simulink model "sampleModel1914"  (R2023a)
settings: Solver=VariableStepAuto  StartTime=0.0  StopTime=10.0  RelTol=1e-3
libraries: hdlsllib x3, simulink x2
settings Model: Creator=user1  LastModifiedBy=user1

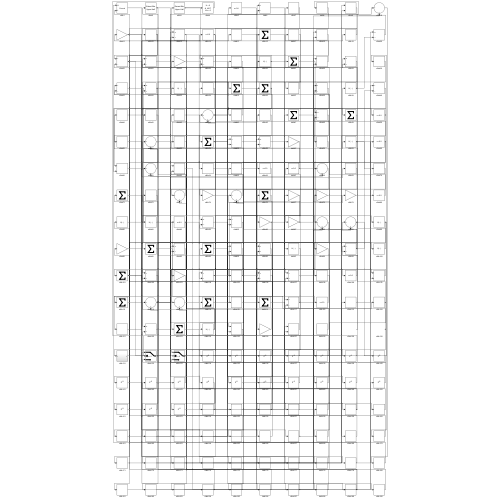
[thumbnail: Simulink's stored preview of the top-level diagram]
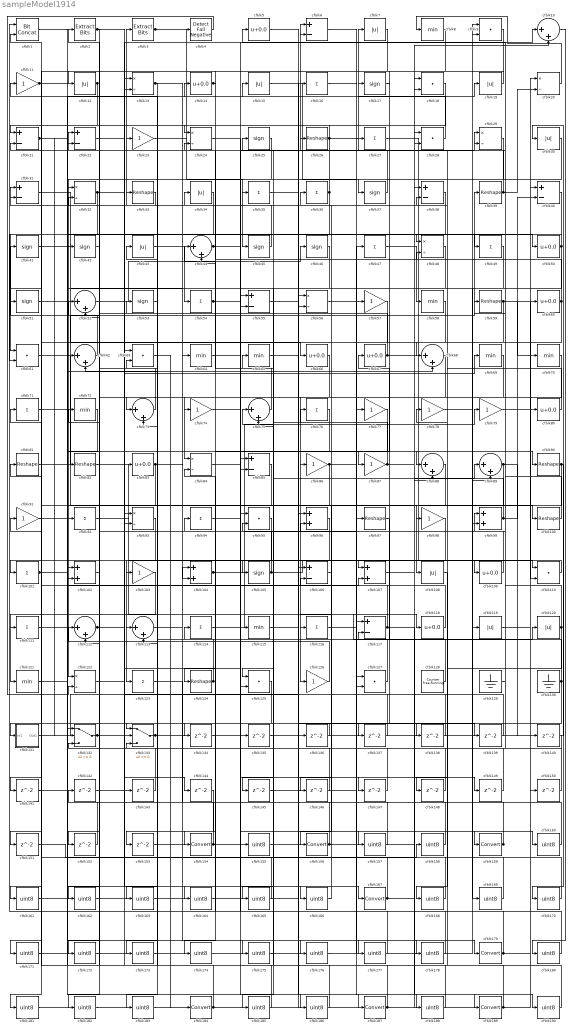
== system sampleModel1914 ==
  cfblk1 : hdlsllib/Logic and Bit Operations/Bit Concat  numInputs=2
  cfblk{10,44,52,62,68,73,75,88..89,112..113} (11 alike) : Sum  Inputs=|++
  cfblk{26,33,39,59,81..82,90,97,100,124} (10 alike) : Reshape
  cfblk{16,27,35..36,47,49,54,71,76,92,94,101,111,114,116,123} (16 alike) : Sum  Inputs=+
  cfblk{96,99,102,104,107} (5 alike) : Sum
  cfblk{11,23,57,74,77..79,86..87,91,98,103,126} (13 alike) : Gain
  cfblk{17,25,37,41..42,45..46,51,53,105} (10 alike) : Signum
  cfblk{6,21..22,31,38,40,55,85,106,117} (10 alike) : Sum  Inputs=+-
  cfblk{7,12,15,19,30,34,43,108,119..120} (10 alike) : Abs  SaturateOnIntegerOverflow=off
  cfblk{5,14,50,60,66..67,80,83,109,118} (10 alike) : Bias  Bias=0.0  SaturateOnIntegerOverflow=off
  cfblk{9,18,28,61,63,95,110,125,127} (9 alike) : DotProduct  OutDataTypeStr=Inherit: Inherit via internal rule
  cfblk{8,58,64..65,69..70,72,115,121} (9 alike) : MinMax
  cfblk{13,20,24,29,32,48,56,84,93,122} (10 alike) : Product  Inputs=*/  RndMeth=Zero  SaturateOnIntegerOverflow=on
  cfblk128 : hdlsllib/Sources/Counter Free-Running  NumBits=16  tsamp=-1
  cfblk129 : Ground
  cfblk130 : Ground
  cfblk131 : Subsystem
      settings: LibrarySourceBlock=|
      | hdlsllib/Ports &
      | Subsystems/Subsystem
  cfblk132 : Switch  SaturateOnIntegerOverflow=off  InputSameDT=off
  cfblk133 : Switch  SaturateOnIntegerOverflow=off  InputSameDT=off
  cfblk{134..153} (20 alike) : Delay  SampleTime=1
  cfblk{154,156,159,167,179,184,187,189} (8 alike) : DataTypeConversion  SaturateOnIntegerOverflow=off  RndMeth=Floor
  cfblk{155,157..158,160..166,168..178,180..183,185..186,188,190} (29 alike) : DataTypeConversion  OutDataTypeStr=uint8  SaturateOnIntegerOverflow=off  RndMeth=Floor
  cfblk2 : simulink/Logic and Bit Operations/Extract Bits  bitsToExtract=Upper half  numBits=8  bitIdxRange=[0 7]  outScalingMode=Preserve fixed-point scaling
      settings: LibrarySourceBlock=|
      | hdlsllib/Logic and Bit
      | Operations/Extract Bits
  cfblk3 : simulink/Logic and Bit Operations/Extract Bits  bitsToExtract=Upper half  numBits=8  bitIdxRange=[0 7]  outScalingMode=Preserve fixed-point scaling
      settings: LibrarySourceBlock=|
      | hdlsllib/Logic and Bit
      | Operations/Extract Bits
  cfblk4 : hdlsllib/Logic and Bit Operations/Detect Fall Negative  vinit=0  OutDataTypeStr=boolean
  wires:
  cfblk83/1 -> cfblk105/1, cfblk182/1
  cfblk105/1 -> cfblk107/1, cfblk72/1
  cfblk86/1 -> cfblk117/1, cfblk151/1
  cfblk19/1 -> cfblk12/1
  cfblk82/1 -> cfblk120/1
  cfblk104/1 -> cfblk79/1, cfblk84/2
  cfblk106/1 -> cfblk156/1
  cfblk130/1 -> cfblk67/1, cfblk183/1
  cfblk66/1 -> cfblk126/1
  cfblk94/1 -> cfblk179/1
  cfblk45/1 -> cfblk3/1
  cfblk46/1 -> cfblk125/1
  cfblk72/1 -> cfblk122/1
  cfblk67/1 -> cfblk109/1, cfblk31/2
  cfblk30/1 -> cfblk45/1
  cfblk103/1 -> cfblk121/1
  cfblk114/1 -> cfblk47/1
  cfblk25/1 -> cfblk92/1
  cfblk37/1 -> cfblk7/1
  cfblk27/1 -> cfblk100/1
  cfblk3/1 -> cfblk35/1, cfblk4/1
  cfblk92/1 -> cfblk110/1
  cfblk99/1 -> cfblk25/1, cfblk24/2, cfblk40/2
  cfblk40/1 -> cfblk61/1
  cfblk5/1 -> cfblk96/1
  cfblk12/1 -> cfblk21/1, cfblk51/1
  cfblk61/1 -> cfblk108/1
  cfblk93/1 -> cfblk123/1
  cfblk20/1 -> cfblk8/1
  cfblk31/1 -> cfblk66/1
  cfblk6/1 -> cfblk27/1
  cfblk73/1 -> cfblk52/1
  cfblk117/1 -> cfblk31/1, cfblk190/1
  cfblk43/1 -> cfblk54/1
  cfblk80/1 -> cfblk34/1
  cfblk81/1 -> cfblk39/1
  cfblk89/1 -> cfblk116/1, cfblk140/1
  cfblk129/1 -> cfblk99/1
  cfblk47/1 -> cfblk58/1
  cfblk23/1 -> cfblk115/1
  cfblk118/1 -> cfblk81/1
  cfblk15/1 -> cfblk97/1
  cfblk95/1 -> cfblk101/1
  cfblk50/1 -> cfblk99/2, cfblk48/1
  cfblk133/1 -> cfblk30/1, cfblk89/2
  cfblk109/1 -> cfblk75/1
  cfblk63/1 -> cfblk184/1
  cfblk21/1 -> cfblk82/1, cfblk132/2
  cfblk26/1 -> cfblk90/1, cfblk24/1, cfblk21/2
  cfblk41/1 -> cfblk64/1
  cfblk52/1 -> cfblk46/1
  cfblk2/1 -> cfblk42/1, cfblk125/2
  cfblk71/1 -> cfblk167/1
  cfblk62/1 -> cfblk41/1
  cfblk28/1 -> cfblk17/1
  cfblk36/1 -> cfblk6/1, cfblk124/1, cfblk103/1
  cfblk39/1 -> cfblk22/1, cfblk20/2
  cfblk121/1 -> cfblk14/1
  cfblk17/1 -> cfblk87/1
  cfblk38/1 -> cfblk55/2
  cfblk32/1 -> cfblk13/1, cfblk111/1
  cfblk126/1 -> cfblk112/1
  cfblk13/1 -> cfblk98/1, cfblk73/1
  cfblk128/1 -> cfblk114/1
  cfblk100/1 -> cfblk5/1
  cfblk110/1 -> cfblk102/1
  cfblk91/1 -> cfblk187/1
  cfblk127/1 -> cfblk117/2
  cfblk87/1 -> cfblk53/1, cfblk10/2
  cfblk11/1 -> cfblk49/1, cfblk86/1
  cfblk101/1 -> cfblk107/2, cfblk166/1
  cfblk64/1 -> cfblk6/2
  cfblk120/1 -> cfblk59/1, cfblk148/1
  cfblk56/1 -> cfblk159/1
  cfblk60/1 -> cfblk22/2, cfblk153/1, cfblk161/1
  cfblk70/1 -> cfblk84/1
  cfblk131/1(Out1) -> cfblk16/1
  cfblk54/1 -> cfblk88/1, cfblk26/1
  cfblk33/1 -> cfblk32/2
  cfblk58/1 -> cfblk68/1
  cfblk112/1 -> cfblk83/1, cfblk69/1, cfblk144/1
  cfblk4/1 -> cfblk122/2
  cfblk51/1 -> cfblk68/2
  cfblk59/1 -> cfblk110/2, cfblk75/2, cfblk70/1
  cfblk65/1 -> cfblk189/1
  cfblk119/1 -> cfblk60/1
  cfblk8/1 -> cfblk37/1
  cfblk79/1 -> cfblk20/1
  cfblk96/1 -> cfblk113/1
  cfblk132/1 -> cfblk15/1, cfblk10/1
  cfblk55/1 -> cfblk29/1
  cfblk42/1 -> cfblk62/1
  cfblk22/1 -> cfblk13/2
  cfblk49/1 -> cfblk102/2
  cfblk34/1 -> cfblk61/2
  cfblk124/1 -> cfblk11/1, cfblk62/2
  cfblk111/1 -> cfblk19/1
  cfblk48/1 -> cfblk104/2
  cfblk107/1 -> cfblk89/1
  cfblk75/1 -> cfblk44/1
  cfblk102/1 -> cfblk112/2
  cfblk44/1 -> cfblk50/1, cfblk149/1
  cfblk125/1 -> cfblk131/1(In1)
  cfblk14/1 -> cfblk74/1, cfblk44/2
  cfblk90/1 -> cfblk146/1, cfblk170/1
  cfblk113/1 -> cfblk118/1
  cfblk57/1 -> cfblk154/1
  cfblk7/1 -> cfblk134/1
  cfblk84/1 -> cfblk135/1
  cfblk136/1 -> cfblk133/1
  cfblk97/1 -> cfblk137/1
  cfblk137/1 -> cfblk113/2
  cfblk115/1 -> cfblk138/1
  cfblk138/1 -> cfblk96/2
  cfblk116/1 -> cfblk139/1
  cfblk139/1 -> cfblk93/1
  cfblk140/1 -> cfblk132/3
  cfblk88/1 -> cfblk141/1
  cfblk122/1 -> cfblk143/1
  cfblk143/1 -> cfblk133/2
  cfblk69/1 -> cfblk145/1
  cfblk145/1 -> cfblk127/2
  cfblk146/1 -> cfblk73/2
  cfblk24/1 -> cfblk147/1
  cfblk147/1 -> cfblk55/1
  cfblk148/1 -> cfblk52/2
  cfblk149/1 -> cfblk38/2
  cfblk150/1 -> cfblk29/2
  cfblk68/1 -> cfblk152/1
  cfblk152/1 -> cfblk32/1
  cfblk153/1 -> cfblk28/2
  cfblk154/1 -> cfblk2/1, cfblk186/1
  cfblk74/1 -> cfblk155/1
  cfblk155/1 -> cfblk57/1
  cfblk156/1 -> cfblk33/1, cfblk36/1
  cfblk35/1 -> cfblk157/1
  cfblk157/1 -> cfblk106/1
  cfblk151/1 -> cfblk158/1
  cfblk158/1 -> cfblk106/2
  cfblk159/1 -> cfblk133/3, cfblk104/1
  cfblk134/1 -> cfblk160/1
  cfblk160/1 -> cfblk56/1
  cfblk161/1 -> cfblk56/2
  cfblk85/1 -> cfblk162/1
  cfblk162/1 -> cfblk93/2
  cfblk53/1 -> cfblk163/1
  cfblk163/1 -> cfblk85/1
  cfblk142/1 -> cfblk164/1
  cfblk164/1 -> cfblk85/2
  cfblk76/1 -> cfblk165/1
  cfblk165/1 -> cfblk23/1
  cfblk166/1 -> cfblk76/1
  cfblk167/1 -> cfblk88/2, cfblk95/2
  cfblk108/1 -> cfblk168/1
  cfblk168/1 -> cfblk71/1
  cfblk78/1 -> cfblk169/1
  cfblk169/1 -> cfblk127/1
  cfblk170/1 -> cfblk78/1
  cfblk9/1 -> cfblk171/1
  cfblk171/1 -> cfblk28/1
  cfblk29/1 -> cfblk172/1
  cfblk172/1 -> cfblk9/1
  cfblk144/1 -> cfblk173/1
  cfblk173/1 -> cfblk9/2
  cfblk77/1 -> cfblk174/1
  cfblk174/1 -> cfblk119/1
  cfblk123/1 -> cfblk175/1
  cfblk175/1 -> cfblk77/1
  cfblk1/1 -> cfblk176/1
  cfblk176/1 -> cfblk38/1
  cfblk135/1 -> cfblk177/1
  cfblk177/1 -> cfblk1/1
  cfblk141/1 -> cfblk178/1
  cfblk178/1 -> cfblk1/2
  cfblk179/1 -> cfblk40/1, cfblk95/1
  cfblk10/1 -> cfblk180/1
  cfblk180/1 -> cfblk94/1
  cfblk18/1 -> cfblk181/1
  cfblk181/1 -> cfblk80/1
  cfblk182/1 -> cfblk18/1
  cfblk183/1 -> cfblk18/2
  cfblk184/1 -> cfblk136/1, cfblk132/1
  cfblk98/1 -> cfblk185/1
  cfblk185/1 -> cfblk63/1
  cfblk186/1 -> cfblk63/2
  cfblk187/1 -> cfblk150/1, cfblk43/1
  cfblk16/1 -> cfblk188/1
  cfblk188/1 -> cfblk91/1
  cfblk189/1 -> cfblk142/1, cfblk48/2
  cfblk190/1 -> cfblk65/1

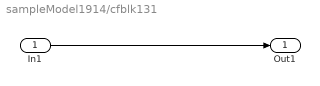
== system sampleModel1914/cfblk131 ==
  In1 : Inport
  Out1 : Outport
  wires:
  In1/1 -> Out1/1
